simulink model "c00006M_harness"  (R2018a)
settings: Solver=FixedStepAuto  StartTime=0.0  StopTime=300  FixedStep=0.1  RelTol=1e-3
undefined symbols (not defined in the file): A1, hmax, PriorityTank, R1, R2, sigbuilder_block, TempThreshold
(part 5 of 66)

== system c00006M_harness/Eval85 ==
  In2 : Inport
  In3 : Inport  Port=2
  Constant1 : Constant
  Data Type Conversion1 : DataTypeConversion
  Data Type Conversion2 : DataTypeConversion
  Memory2 : Memory  InitialCondition=1
  Memory3 : Memory  InitialCondition=1
  MinMax : MinMax  Inputs=3
  MinMax2 : MinMax  Inputs=2
  MinMax3 : MinMax  Inputs=2
  ROOut2 : RelationalOperator  Operator===  OutDataTypeStr=boolean  RndMeth=Simplest
  ROOut3 : RelationalOperator  Operator===  OutDataTypeStr=boolean  RndMeth=Simplest
  Out1 : Outport
  wires:
  Data Type Conversion2/1 -> MinMax3/1
  Data Type Conversion1/1 -> MinMax2/1
  MinMax2/1 -> MinMax/2, Memory2/1
  Memory2/1 -> MinMax2/2
  Memory3/1 -> MinMax3/2
  ROOut2/1 -> Data Type Conversion1/1
  ROOut3/1 -> Data Type Conversion2/1
  MinMax3/1 -> Memory3/1, MinMax/3
  [out2] -> ROOut2/2
  In2/1 -> ROOut2/1
  In3/1 -> ROOut3/1
  [out3] -> ROOut3/2
  MinMax/1 -> Out1/1
  Constant1/1 -> MinMax/1

== system c00006M_harness/Eval86 ==
  In2 : Inport
  In3 : Inport  Port=2
  Constant1 : Constant
  Data Type Conversion1 : DataTypeConversion
  Data Type Conversion2 : DataTypeConversion
  Memory2 : Memory  InitialCondition=1
  Memory3 : Memory  InitialCondition=1
  MinMax : MinMax  Inputs=3
  MinMax2 : MinMax  Inputs=2
  MinMax3 : MinMax  Inputs=2
  ROOut2 : RelationalOperator  Operator===  OutDataTypeStr=boolean  RndMeth=Simplest
  ROOut3 : RelationalOperator  Operator===  OutDataTypeStr=boolean  RndMeth=Simplest
  Out1 : Outport
  wires:
  Data Type Conversion2/1 -> MinMax3/1
  Data Type Conversion1/1 -> MinMax2/1
  MinMax2/1 -> MinMax/2, Memory2/1
  Memory2/1 -> MinMax2/2
  Memory3/1 -> MinMax3/2
  ROOut2/1 -> Data Type Conversion1/1
  ROOut3/1 -> Data Type Conversion2/1
  MinMax3/1 -> Memory3/1, MinMax/3
  [out2] -> ROOut2/2
  In2/1 -> ROOut2/1
  In3/1 -> ROOut3/1
  [out3] -> ROOut3/2
  MinMax/1 -> Out1/1
  Constant1/1 -> MinMax/1

== system c00006M_harness/Eval87 ==
  In2 : Inport
  In3 : Inport  Port=2
  Constant1 : Constant
  Data Type Conversion1 : DataTypeConversion
  Data Type Conversion2 : DataTypeConversion
  Memory2 : Memory  InitialCondition=1
  Memory3 : Memory  InitialCondition=1
  MinMax : MinMax  Inputs=3
  MinMax2 : MinMax  Inputs=2
  MinMax3 : MinMax  Inputs=2
  ROOut2 : RelationalOperator  Operator===  OutDataTypeStr=boolean  RndMeth=Simplest
  ROOut3 : RelationalOperator  Operator===  OutDataTypeStr=boolean  RndMeth=Simplest
  Out1 : Outport
  wires:
  Data Type Conversion2/1 -> MinMax3/1
  Data Type Conversion1/1 -> MinMax2/1
  MinMax2/1 -> MinMax/2, Memory2/1
  Memory2/1 -> MinMax2/2
  Memory3/1 -> MinMax3/2
  ROOut2/1 -> Data Type Conversion1/1
  ROOut3/1 -> Data Type Conversion2/1
  MinMax3/1 -> Memory3/1, MinMax/3
  [out2] -> ROOut2/2
  In2/1 -> ROOut2/1
  In3/1 -> ROOut3/1
  [out3] -> ROOut3/2
  MinMax/1 -> Out1/1
  Constant1/1 -> MinMax/1

== system c00006M_harness/Eval88 ==
  In2 : Inport
  In3 : Inport  Port=2
  Constant1 : Constant
  Data Type Conversion1 : DataTypeConversion
  Data Type Conversion2 : DataTypeConversion
  Memory2 : Memory  InitialCondition=1
  Memory3 : Memory  InitialCondition=1
  MinMax : MinMax  Inputs=3
  MinMax2 : MinMax  Inputs=2
  MinMax3 : MinMax  Inputs=2
  ROOut2 : RelationalOperator  Operator===  OutDataTypeStr=boolean  RndMeth=Simplest
  ROOut3 : RelationalOperator  Operator===  OutDataTypeStr=boolean  RndMeth=Simplest
  Out1 : Outport
  wires:
  Data Type Conversion2/1 -> MinMax3/1
  Data Type Conversion1/1 -> MinMax2/1
  MinMax2/1 -> MinMax/2, Memory2/1
  Memory2/1 -> MinMax2/2
  Memory3/1 -> MinMax3/2
  ROOut2/1 -> Data Type Conversion1/1
  ROOut3/1 -> Data Type Conversion2/1
  MinMax3/1 -> Memory3/1, MinMax/3
  [out2] -> ROOut2/2
  In2/1 -> ROOut2/1
  In3/1 -> ROOut3/1
  [out3] -> ROOut3/2
  MinMax/1 -> Out1/1
  Constant1/1 -> MinMax/1

== system c00006M_harness/Eval89 ==
  In2 : Inport
  In3 : Inport  Port=2
  Constant1 : Constant
  Data Type Conversion1 : DataTypeConversion
  Data Type Conversion2 : DataTypeConversion
  Memory2 : Memory  InitialCondition=1
  Memory3 : Memory  InitialCondition=1
  MinMax : MinMax  Inputs=3
  MinMax2 : MinMax  Inputs=2
  MinMax3 : MinMax  Inputs=2
  ROOut2 : RelationalOperator  Operator===  OutDataTypeStr=boolean  RndMeth=Simplest
  ROOut3 : RelationalOperator  Operator===  OutDataTypeStr=boolean  RndMeth=Simplest
  Out1 : Outport
  wires:
  Data Type Conversion2/1 -> MinMax3/1
  Data Type Conversion1/1 -> MinMax2/1
  MinMax2/1 -> MinMax/2, Memory2/1
  Memory2/1 -> MinMax2/2
  Memory3/1 -> MinMax3/2
  ROOut2/1 -> Data Type Conversion1/1
  ROOut3/1 -> Data Type Conversion2/1
  MinMax3/1 -> Memory3/1, MinMax/3
  [out2] -> ROOut2/2
  In2/1 -> ROOut2/1
  In3/1 -> ROOut3/1
  [out3] -> ROOut3/2
  MinMax/1 -> Out1/1
  Constant1/1 -> MinMax/1

== system c00006M_harness/Eval90 ==
  In2 : Inport
  In3 : Inport  Port=2
  Constant1 : Constant
  Data Type Conversion1 : DataTypeConversion
  Data Type Conversion2 : DataTypeConversion
  Memory2 : Memory  InitialCondition=1
  Memory3 : Memory  InitialCondition=1
  MinMax : MinMax  Inputs=3
  MinMax2 : MinMax  Inputs=2
  MinMax3 : MinMax  Inputs=2
  ROOut2 : RelationalOperator  Operator===  OutDataTypeStr=boolean  RndMeth=Simplest
  ROOut3 : RelationalOperator  Operator===  OutDataTypeStr=boolean  RndMeth=Simplest
  Out1 : Outport
  wires:
  Data Type Conversion2/1 -> MinMax3/1
  Data Type Conversion1/1 -> MinMax2/1
  MinMax2/1 -> MinMax/2, Memory2/1
  Memory2/1 -> MinMax2/2
  Memory3/1 -> MinMax3/2
  ROOut2/1 -> Data Type Conversion1/1
  ROOut3/1 -> Data Type Conversion2/1
  MinMax3/1 -> Memory3/1, MinMax/3
  [out2] -> ROOut2/2
  In2/1 -> ROOut2/1
  In3/1 -> ROOut3/1
  [out3] -> ROOut3/2
  MinMax/1 -> Out1/1
  Constant1/1 -> MinMax/1

== system c00006M_harness/Eval91 ==
  In2 : Inport
  In3 : Inport  Port=2
  Constant1 : Constant
  Data Type Conversion1 : DataTypeConversion
  Data Type Conversion2 : DataTypeConversion
  Memory2 : Memory  InitialCondition=1
  Memory3 : Memory  InitialCondition=1
  MinMax : MinMax  Inputs=3
  MinMax2 : MinMax  Inputs=2
  MinMax3 : MinMax  Inputs=2
  ROOut2 : RelationalOperator  Operator===  OutDataTypeStr=boolean  RndMeth=Simplest
  ROOut3 : RelationalOperator  Operator===  OutDataTypeStr=boolean  RndMeth=Simplest
  Out1 : Outport
  wires:
  Data Type Conversion2/1 -> MinMax3/1
  Data Type Conversion1/1 -> MinMax2/1
  MinMax2/1 -> MinMax/2, Memory2/1
  Memory2/1 -> MinMax2/2
  Memory3/1 -> MinMax3/2
  ROOut2/1 -> Data Type Conversion1/1
  ROOut3/1 -> Data Type Conversion2/1
  MinMax3/1 -> Memory3/1, MinMax/3
  [out2] -> ROOut2/2
  In2/1 -> ROOut2/1
  In3/1 -> ROOut3/1
  [out3] -> ROOut3/2
  MinMax/1 -> Out1/1
  Constant1/1 -> MinMax/1

== system c00006M_harness/Eval92 ==
  In2 : Inport
  In3 : Inport  Port=2
  Constant1 : Constant
  Data Type Conversion1 : DataTypeConversion
  Data Type Conversion2 : DataTypeConversion
  Memory2 : Memory  InitialCondition=1
  Memory3 : Memory  InitialCondition=1
  MinMax : MinMax  Inputs=3
  MinMax2 : MinMax  Inputs=2
  MinMax3 : MinMax  Inputs=2
  ROOut2 : RelationalOperator  Operator===  OutDataTypeStr=boolean  RndMeth=Simplest
  ROOut3 : RelationalOperator  Operator===  OutDataTypeStr=boolean  RndMeth=Simplest
  Out1 : Outport
  wires:
  Data Type Conversion2/1 -> MinMax3/1
  Data Type Conversion1/1 -> MinMax2/1
  MinMax2/1 -> MinMax/2, Memory2/1
  Memory2/1 -> MinMax2/2
  Memory3/1 -> MinMax3/2
  ROOut2/1 -> Data Type Conversion1/1
  ROOut3/1 -> Data Type Conversion2/1
  MinMax3/1 -> Memory3/1, MinMax/3
  [out2] -> ROOut2/2
  In2/1 -> ROOut2/1
  In3/1 -> ROOut3/1
  [out3] -> ROOut3/2
  MinMax/1 -> Out1/1
  Constant1/1 -> MinMax/1

== system c00006M_harness/Eval93 ==
  In2 : Inport
  In3 : Inport  Port=2
  Constant1 : Constant
  Data Type Conversion1 : DataTypeConversion
  Data Type Conversion2 : DataTypeConversion
  Memory2 : Memory  InitialCondition=1
  Memory3 : Memory  InitialCondition=1
  MinMax : MinMax  Inputs=3
  MinMax2 : MinMax  Inputs=2
  MinMax3 : MinMax  Inputs=2
  ROOut2 : RelationalOperator  Operator===  OutDataTypeStr=boolean  RndMeth=Simplest
  ROOut3 : RelationalOperator  Operator===  OutDataTypeStr=boolean  RndMeth=Simplest
  Out1 : Outport
  wires:
  Data Type Conversion2/1 -> MinMax3/1
  Data Type Conversion1/1 -> MinMax2/1
  MinMax2/1 -> MinMax/2, Memory2/1
  Memory2/1 -> MinMax2/2
  Memory3/1 -> MinMax3/2
  ROOut2/1 -> Data Type Conversion1/1
  ROOut3/1 -> Data Type Conversion2/1
  MinMax3/1 -> Memory3/1, MinMax/3
  [out2] -> ROOut2/2
  In2/1 -> ROOut2/1
  In3/1 -> ROOut3/1
  [out3] -> ROOut3/2
  MinMax/1 -> Out1/1
  Constant1/1 -> MinMax/1

== system c00006M_harness/Eval94 ==
  In2 : Inport
  In3 : Inport  Port=2
  Constant1 : Constant
  Data Type Conversion1 : DataTypeConversion
  Data Type Conversion2 : DataTypeConversion
  Memory2 : Memory  InitialCondition=1
  Memory3 : Memory  InitialCondition=1
  MinMax : MinMax  Inputs=3
  MinMax2 : MinMax  Inputs=2
  MinMax3 : MinMax  Inputs=2
  ROOut2 : RelationalOperator  Operator===  OutDataTypeStr=boolean  RndMeth=Simplest
  ROOut3 : RelationalOperator  Operator===  OutDataTypeStr=boolean  RndMeth=Simplest
  Out1 : Outport
  wires:
  Data Type Conversion2/1 -> MinMax3/1
  Data Type Conversion1/1 -> MinMax2/1
  MinMax2/1 -> MinMax/2, Memory2/1
  Memory2/1 -> MinMax2/2
  Memory3/1 -> MinMax3/2
  ROOut2/1 -> Data Type Conversion1/1
  ROOut3/1 -> Data Type Conversion2/1
  MinMax3/1 -> Memory3/1, MinMax/3
  [out2] -> ROOut2/2
  In2/1 -> ROOut2/1
  In3/1 -> ROOut3/1
  [out3] -> ROOut3/2
  MinMax/1 -> Out1/1
  Constant1/1 -> MinMax/1

== system c00006M_harness/Eval95 ==
  In2 : Inport
  In3 : Inport  Port=2
  Constant1 : Constant
  Data Type Conversion1 : DataTypeConversion
  Data Type Conversion2 : DataTypeConversion
  Memory2 : Memory  InitialCondition=1
  Memory3 : Memory  InitialCondition=1
  MinMax : MinMax  Inputs=3
  MinMax2 : MinMax  Inputs=2
  MinMax3 : MinMax  Inputs=2
  ROOut2 : RelationalOperator  Operator===  OutDataTypeStr=boolean  RndMeth=Simplest
  ROOut3 : RelationalOperator  Operator===  OutDataTypeStr=boolean  RndMeth=Simplest
  Out1 : Outport
  wires:
  Data Type Conversion2/1 -> MinMax3/1
  Data Type Conversion1/1 -> MinMax2/1
  MinMax2/1 -> MinMax/2, Memory2/1
  Memory2/1 -> MinMax2/2
  Memory3/1 -> MinMax3/2
  ROOut2/1 -> Data Type Conversion1/1
  ROOut3/1 -> Data Type Conversion2/1
  MinMax3/1 -> Memory3/1, MinMax/3
  [out2] -> ROOut2/2
  In2/1 -> ROOut2/1
  In3/1 -> ROOut3/1
  [out3] -> ROOut3/2
  MinMax/1 -> Out1/1
  Constant1/1 -> MinMax/1

== system c00006M_harness/Eval96 ==
  In2 : Inport
  In3 : Inport  Port=2
  Constant1 : Constant
  Data Type Conversion1 : DataTypeConversion
  Data Type Conversion2 : DataTypeConversion
  Memory2 : Memory  InitialCondition=1
  Memory3 : Memory  InitialCondition=1
  MinMax : MinMax  Inputs=3
  MinMax2 : MinMax  Inputs=2
  MinMax3 : MinMax  Inputs=2
  ROOut2 : RelationalOperator  Operator===  OutDataTypeStr=boolean  RndMeth=Simplest
  ROOut3 : RelationalOperator  Operator===  OutDataTypeStr=boolean  RndMeth=Simplest
  Out1 : Outport
  wires:
  Data Type Conversion2/1 -> MinMax3/1
  Data Type Conversion1/1 -> MinMax2/1
  MinMax2/1 -> MinMax/2, Memory2/1
  Memory2/1 -> MinMax2/2
  Memory3/1 -> MinMax3/2
  ROOut2/1 -> Data Type Conversion1/1
  ROOut3/1 -> Data Type Conversion2/1
  MinMax3/1 -> Memory3/1, MinMax/3
  [out2] -> ROOut2/2
  In2/1 -> ROOut2/1
  In3/1 -> ROOut3/1
  [out3] -> ROOut3/2
  MinMax/1 -> Out1/1
  Constant1/1 -> MinMax/1

== system c00006M_harness/Eval97 ==
  In2 : Inport
  In3 : Inport  Port=2
  Constant1 : Constant
  Data Type Conversion1 : DataTypeConversion
  Data Type Conversion2 : DataTypeConversion
  Memory2 : Memory  InitialCondition=1
  Memory3 : Memory  InitialCondition=1
  MinMax : MinMax  Inputs=3
  MinMax2 : MinMax  Inputs=2
  MinMax3 : MinMax  Inputs=2
  ROOut2 : RelationalOperator  Operator===  OutDataTypeStr=boolean  RndMeth=Simplest
  ROOut3 : RelationalOperator  Operator===  OutDataTypeStr=boolean  RndMeth=Simplest
  Out1 : Outport
  wires:
  Data Type Conversion2/1 -> MinMax3/1
  Data Type Conversion1/1 -> MinMax2/1
  MinMax2/1 -> MinMax/2, Memory2/1
  Memory2/1 -> MinMax2/2
  Memory3/1 -> MinMax3/2
  ROOut2/1 -> Data Type Conversion1/1
  ROOut3/1 -> Data Type Conversion2/1
  MinMax3/1 -> Memory3/1, MinMax/3
  [out2] -> ROOut2/2
  In2/1 -> ROOut2/1
  In3/1 -> ROOut3/1
  [out3] -> ROOut3/2
  MinMax/1 -> Out1/1
  Constant1/1 -> MinMax/1

== system c00006M_harness/Eval98 ==
  In2 : Inport
  In3 : Inport  Port=2
  Constant1 : Constant
  Data Type Conversion1 : DataTypeConversion
  Data Type Conversion2 : DataTypeConversion
  Memory2 : Memory  InitialCondition=1
  Memory3 : Memory  InitialCondition=1
  MinMax : MinMax  Inputs=3
  MinMax2 : MinMax  Inputs=2
  MinMax3 : MinMax  Inputs=2
  ROOut2 : RelationalOperator  Operator===  OutDataTypeStr=boolean  RndMeth=Simplest
  ROOut3 : RelationalOperator  Operator===  OutDataTypeStr=boolean  RndMeth=Simplest
  Out1 : Outport
  wires:
  Data Type Conversion2/1 -> MinMax3/1
  Data Type Conversion1/1 -> MinMax2/1
  MinMax2/1 -> MinMax/2, Memory2/1
  Memory2/1 -> MinMax2/2
  Memory3/1 -> MinMax3/2
  ROOut2/1 -> Data Type Conversion1/1
  ROOut3/1 -> Data Type Conversion2/1
  MinMax3/1 -> Memory3/1, MinMax/3
  [out2] -> ROOut2/2
  In2/1 -> ROOut2/1
  In3/1 -> ROOut3/1
  [out3] -> ROOut3/2
  MinMax/1 -> Out1/1
  Constant1/1 -> MinMax/1

== system c00006M_harness/Eval99 ==
  In2 : Inport
  In3 : Inport  Port=2
  Constant1 : Constant
  Data Type Conversion1 : DataTypeConversion
  Data Type Conversion2 : DataTypeConversion
  Memory2 : Memory  InitialCondition=1
  Memory3 : Memory  InitialCondition=1
  MinMax : MinMax  Inputs=3
  MinMax2 : MinMax  Inputs=2
  MinMax3 : MinMax  Inputs=2
  ROOut2 : RelationalOperator  Operator===  OutDataTypeStr=boolean  RndMeth=Simplest
  ROOut3 : RelationalOperator  Operator===  OutDataTypeStr=boolean  RndMeth=Simplest
  Out1 : Outport
  wires:
  Data Type Conversion2/1 -> MinMax3/1
  Data Type Conversion1/1 -> MinMax2/1
  MinMax2/1 -> MinMax/2, Memory2/1
  Memory2/1 -> MinMax2/2
  Memory3/1 -> MinMax3/2
  ROOut2/1 -> Data Type Conversion1/1
  ROOut3/1 -> Data Type Conversion2/1
  MinMax3/1 -> Memory3/1, MinMax/3
  [out2] -> ROOut2/2
  In2/1 -> ROOut2/1
  In3/1 -> ROOut3/1
  [out3] -> ROOut3/2
  MinMax/1 -> Out1/1
  Constant1/1 -> MinMax/1

== system c00006M_harness/Inputs ==
  Demux : Demux  Tag=STV Demux  Outputs=12
  FromWs : FromWorkspace  Tag=STV FromWs  VariableName=tuvar  SampleTime=0
  CT2 : Outport  Tag=STV Outport
  F2 : Outport  Tag=STV Outport  Port=2
  E2 : Outport  Tag=STV Outport  Port=3
  MR2 : Outport  Tag=STV Outport  Port=4
  T2 : Outport  Tag=STV Outport  Port=5
  EB2 : Outport  Tag=STV Outport  Port=6
  CT3 : Outport  Tag=STV Outport  Port=7
  F3 : Outport  Tag=STV Outport  Port=8
  E3 : Outport  Tag=STV Outport  Port=9
  MR3 : Outport  Tag=STV Outport  Port=10
  T3 : Outport  Tag=STV Outport  Port=11
  EB3 : Outport  Tag=STV Outport  Port=12
  wires:
  Demux/12 -> EB3/1
  Demux/11 -> T3/1
  Demux/10 -> MR3/1
  Demux/9 -> E3/1
  Demux/8 -> F3/1
  Demux/7 -> CT3/1
  Demux/6 -> EB2/1
  Demux/5 -> T2/1
  Demux/4 -> MR2/1
  Demux/3 -> E2/1
  Demux/2 -> F2/1
  Demux/1 -> CT2/1
  FromWs/1 -> Demux/1

== system c00006M_harness/M062 ==
  note: VALUES
      | ---------------------------------
      | ControlType = 1 | 2 | 3
      | FillTank = 0 | 1
      | EmptyTank = 0 | 1
      | ManualReference between 0 and 1
      | Tempreature between 0 and 100
      | EmergencyButton = 0 | 1
      | LiquidLevel between 0 and 1 (hmax)
  note: Inputs For Tank2
  note: NAMES
      | --------------------------------------------
      | CT1 = ControlType Tank 1
      | F1 = Fill Tank 1
      | E1 = Empty Tank 1
      | MR1 = Manual Reference Tank1
      | T1 = Temperature Tank 1
      | EB1 = Emergency Button Tank 1
      | LL1 = Liquid Level 1
  note: Inputs For Tank3
  note: Inputs For Tank1
  CT2 : Inport
  F2 : Inport  Port=2
  E2 : Inport  Port=3
  MR2 : Inport  Port=4
  T2 : Inport  Port=5
  EB2 : Inport  Port=6
  CT3 : Inport  Port=7
  F3 : Inport  Port=8
  E3 : Inport  Port=9
  MR3 : Inport  Port=10
  T3 : Inport  Port=11
  EB3 : Inport  Port=12
  Tank2 : Subsystem
  Tank3 : Subsystem
  LL2 : Outport
  LL3 : Outport  Port=2
  wires:
  Tank2/1(LL2) -> LL2/1, Tank3/7(LL2)
  Tank3/1(LL3) -> LL3/1, Tank2/7(LL3)
  EB2/1 -> Tank2/6(EB2)
  MR3/1 -> Tank3/4(MR3)
  CT2/1 -> Tank2/1(CT2)
  F2/1 -> Tank2/2(F2)
  E3/1 -> Tank3/3(E3)
  E2/1 -> Tank2/3(E2)
  T2/1 -> Tank2/5(T2)
  CT3/1 -> Tank3/1(CT3)
  F3/1 -> Tank3/2(F3)
  EB3/1 -> Tank3/6(EB3)
  T3/1 -> Tank3/5(T3)
  MR2/1 -> Tank2/4(MR2)

== system c00006M_harness/M063 ==
  note: VALUES
      | ---------------------------------
      | ControlType = 1 | 2 | 3
      | FillTank = 0 | 1
      | EmptyTank = 0 | 1
      | ManualReference between 0 and 1
      | Tempreature between 0 and 100
      | EmergencyButton = 0 | 1
      | LiquidLevel between 0 and 1 (hmax)
  note: Inputs For Tank2
  note: NAMES
      | --------------------------------------------
      | CT1 = ControlType Tank 1
      | F1 = Fill Tank 1
      | E1 = Empty Tank 1
      | MR1 = Manual Reference Tank1
      | T1 = Temperature Tank 1
      | EB1 = Emergency Button Tank 1
      | LL1 = Liquid Level 1
  note: Inputs For Tank3
  note: Inputs For Tank1
  CT2 : Inport
  F2 : Inport  Port=2
  E2 : Inport  Port=3
  MR2 : Inport  Port=4
  T2 : Inport  Port=5
  EB2 : Inport  Port=6
  CT3 : Inport  Port=7
  F3 : Inport  Port=8
  E3 : Inport  Port=9
  MR3 : Inport  Port=10
  T3 : Inport  Port=11
  EB3 : Inport  Port=12
  Tank2 : Subsystem
  Tank3 : Subsystem
  LL2 : Outport
  LL3 : Outport  Port=2
  wires:
  Tank2/1(LL2) -> LL2/1, Tank3/7(LL2)
  Tank3/1(LL3) -> LL3/1, Tank2/7(LL3)
  EB2/1 -> Tank2/6(EB2)
  MR3/1 -> Tank3/4(MR3)
  CT2/1 -> Tank2/1(CT2)
  F2/1 -> Tank2/2(F2)
  E3/1 -> Tank3/3(E3)
  E2/1 -> Tank2/3(E2)
  T2/1 -> Tank2/5(T2)
  CT3/1 -> Tank3/1(CT3)
  F3/1 -> Tank3/2(F3)
  EB3/1 -> Tank3/6(EB3)
  T3/1 -> Tank3/5(T3)
  MR2/1 -> Tank2/4(MR2)

== system c00006M_harness/M064 ==
  note: VALUES
      | ---------------------------------
      | ControlType = 1 | 2 | 3
      | FillTank = 0 | 1
      | EmptyTank = 0 | 1
      | ManualReference between 0 and 1
      | Tempreature between 0 and 100
      | EmergencyButton = 0 | 1
      | LiquidLevel between 0 and 1 (hmax)
  note: Inputs For Tank2
  note: NAMES
      | --------------------------------------------
      | CT1 = ControlType Tank 1
      | F1 = Fill Tank 1
      | E1 = Empty Tank 1
      | MR1 = Manual Reference Tank1
      | T1 = Temperature Tank 1
      | EB1 = Emergency Button Tank 1
      | LL1 = Liquid Level 1
  note: Inputs For Tank3
  note: Inputs For Tank1
  CT2 : Inport
  F2 : Inport  Port=2
  E2 : Inport  Port=3
  MR2 : Inport  Port=4
  T2 : Inport  Port=5
  EB2 : Inport  Port=6
  CT3 : Inport  Port=7
  F3 : Inport  Port=8
  E3 : Inport  Port=9
  MR3 : Inport  Port=10
  T3 : Inport  Port=11
  EB3 : Inport  Port=12
  Tank2 : Subsystem
  Tank3 : Subsystem
  LL2 : Outport
  LL3 : Outport  Port=2
  wires:
  Tank2/1(LL2) -> LL2/1, Tank3/7(LL2)
  Tank3/1(LL3) -> LL3/1, Tank2/7(LL3)
  EB2/1 -> Tank2/6(EB2)
  MR3/1 -> Tank3/4(MR3)
  CT2/1 -> Tank2/1(CT2)
  F2/1 -> Tank2/2(F2)
  E3/1 -> Tank3/3(E3)
  E2/1 -> Tank2/3(E2)
  T2/1 -> Tank2/5(T2)
  CT3/1 -> Tank3/1(CT3)
  F3/1 -> Tank3/2(F3)
  EB3/1 -> Tank3/6(EB3)
  T3/1 -> Tank3/5(T3)
  MR2/1 -> Tank2/4(MR2)

== system c00006M_harness/M065 ==
  note: VALUES
      | ---------------------------------
      | ControlType = 1 | 2 | 3
      | FillTank = 0 | 1
      | EmptyTank = 0 | 1
      | ManualReference between 0 and 1
      | Tempreature between 0 and 100
      | EmergencyButton = 0 | 1
      | LiquidLevel between 0 and 1 (hmax)
  note: Inputs For Tank2
  note: NAMES
      | --------------------------------------------
      | CT1 = ControlType Tank 1
      | F1 = Fill Tank 1
      | E1 = Empty Tank 1
      | MR1 = Manual Reference Tank1
      | T1 = Temperature Tank 1
      | EB1 = Emergency Button Tank 1
      | LL1 = Liquid Level 1
  note: Inputs For Tank3
  note: Inputs For Tank1
  CT2 : Inport
  F2 : Inport  Port=2
  E2 : Inport  Port=3
  MR2 : Inport  Port=4
  T2 : Inport  Port=5
  EB2 : Inport  Port=6
  CT3 : Inport  Port=7
  F3 : Inport  Port=8
  E3 : Inport  Port=9
  MR3 : Inport  Port=10
  T3 : Inport  Port=11
  EB3 : Inport  Port=12
  Tank2 : Subsystem
  Tank3 : Subsystem
  LL2 : Outport
  LL3 : Outport  Port=2
  wires:
  Tank2/1(LL2) -> LL2/1, Tank3/7(LL2)
  Tank3/1(LL3) -> LL3/1, Tank2/7(LL3)
  EB2/1 -> Tank2/6(EB2)
  MR3/1 -> Tank3/4(MR3)
  CT2/1 -> Tank2/1(CT2)
  F2/1 -> Tank2/2(F2)
  E3/1 -> Tank3/3(E3)
  E2/1 -> Tank2/3(E2)
  T2/1 -> Tank2/5(T2)
  CT3/1 -> Tank3/1(CT3)
  F3/1 -> Tank3/2(F3)
  EB3/1 -> Tank3/6(EB3)
  T3/1 -> Tank3/5(T3)
  MR2/1 -> Tank2/4(MR2)

== system c00006M_harness/M066 ==
  note: VALUES
      | ---------------------------------
      | ControlType = 1 | 2 | 3
      | FillTank = 0 | 1
      | EmptyTank = 0 | 1
      | ManualReference between 0 and 1
      | Tempreature between 0 and 100
      | EmergencyButton = 0 | 1
      | LiquidLevel between 0 and 1 (hmax)
  note: Inputs For Tank2
  note: NAMES
      | --------------------------------------------
      | CT1 = ControlType Tank 1
      | F1 = Fill Tank 1
      | E1 = Empty Tank 1
      | MR1 = Manual Reference Tank1
      | T1 = Temperature Tank 1
      | EB1 = Emergency Button Tank 1
      | LL1 = Liquid Level 1
  note: Inputs For Tank3
  note: Inputs For Tank1
  CT2 : Inport
  F2 : Inport  Port=2
  E2 : Inport  Port=3
  MR2 : Inport  Port=4
  T2 : Inport  Port=5
  EB2 : Inport  Port=6
  CT3 : Inport  Port=7
  F3 : Inport  Port=8
  E3 : Inport  Port=9
  MR3 : Inport  Port=10
  T3 : Inport  Port=11
  EB3 : Inport  Port=12
  Tank2 : Subsystem
  Tank3 : Subsystem
  LL2 : Outport
  LL3 : Outport  Port=2
  wires:
  Tank2/1(LL2) -> LL2/1, Tank3/7(LL2)
  Tank3/1(LL3) -> LL3/1, Tank2/7(LL3)
  EB2/1 -> Tank2/6(EB2)
  MR3/1 -> Tank3/4(MR3)
  CT2/1 -> Tank2/1(CT2)
  F2/1 -> Tank2/2(F2)
  E3/1 -> Tank3/3(E3)
  E2/1 -> Tank2/3(E2)
  T2/1 -> Tank2/5(T2)
  CT3/1 -> Tank3/1(CT3)
  F3/1 -> Tank3/2(F3)
  EB3/1 -> Tank3/6(EB3)
  T3/1 -> Tank3/5(T3)
  MR2/1 -> Tank2/4(MR2)

== system c00006M_harness/M083 ==
  note: VALUES
      | ---------------------------------
      | ControlType = 1 | 2 | 3
      | FillTank = 0 | 1
      | EmptyTank = 0 | 1
      | ManualReference between 0 and 1
      | Tempreature between 0 and 100
      | EmergencyButton = 0 | 1
      | LiquidLevel between 0 and 1 (hmax)
  note: Inputs For Tank2
  note: NAMES
      | --------------------------------------------
      | CT1 = ControlType Tank 1
      | F1 = Fill Tank 1
      | E1 = Empty Tank 1
      | MR1 = Manual Reference Tank1
      | T1 = Temperature Tank 1
      | EB1 = Emergency Button Tank 1
      | LL1 = Liquid Level 1
  note: Inputs For Tank3
  note: Inputs For Tank1
  CT2 : Inport
  F2 : Inport  Port=2
  E2 : Inport  Port=3
  MR2 : Inport  Port=4
  T2 : Inport  Port=5
  EB2 : Inport  Port=6
  CT3 : Inport  Port=7
  F3 : Inport  Port=8
  E3 : Inport  Port=9
  MR3 : Inport  Port=10
  T3 : Inport  Port=11
  EB3 : Inport  Port=12
  Tank2 : Subsystem
  Tank3 : Subsystem
  LL2 : Outport
  LL3 : Outport  Port=2
  wires:
  Tank2/1(LL2) -> LL2/1, Tank3/7(LL2)
  Tank3/1(LL3) -> LL3/1, Tank2/7(LL3)
  EB2/1 -> Tank2/6(EB2)
  MR3/1 -> Tank3/4(MR3)
  CT2/1 -> Tank2/1(CT2)
  F2/1 -> Tank2/2(F2)
  E3/1 -> Tank3/3(E3)
  E2/1 -> Tank2/3(E2)
  T2/1 -> Tank2/5(T2)
  CT3/1 -> Tank3/1(CT3)
  F3/1 -> Tank3/2(F3)
  EB3/1 -> Tank3/6(EB3)
  T3/1 -> Tank3/5(T3)
  MR2/1 -> Tank2/4(MR2)

== system c00006M_harness/M084 ==
  note: VALUES
      | ---------------------------------
      | ControlType = 1 | 2 | 3
      | FillTank = 0 | 1
      | EmptyTank = 0 | 1
      | ManualReference between 0 and 1
      | Tempreature between 0 and 100
      | EmergencyButton = 0 | 1
      | LiquidLevel between 0 and 1 (hmax)
  note: Inputs For Tank2
  note: NAMES
      | --------------------------------------------
      | CT1 = ControlType Tank 1
      | F1 = Fill Tank 1
      | E1 = Empty Tank 1
      | MR1 = Manual Reference Tank1
      | T1 = Temperature Tank 1
      | EB1 = Emergency Button Tank 1
      | LL1 = Liquid Level 1
  note: Inputs For Tank3
  note: Inputs For Tank1
  CT2 : Inport
  F2 : Inport  Port=2
  E2 : Inport  Port=3
  MR2 : Inport  Port=4
  T2 : Inport  Port=5
  EB2 : Inport  Port=6
  CT3 : Inport  Port=7
  F3 : Inport  Port=8
  E3 : Inport  Port=9
  MR3 : Inport  Port=10
  T3 : Inport  Port=11
  EB3 : Inport  Port=12
  Tank2 : Subsystem
  Tank3 : Subsystem
  LL2 : Outport
  LL3 : Outport  Port=2
  wires:
  Tank2/1(LL2) -> LL2/1, Tank3/7(LL2)
  Tank3/1(LL3) -> LL3/1, Tank2/7(LL3)
  EB2/1 -> Tank2/6(EB2)
  MR3/1 -> Tank3/4(MR3)
  CT2/1 -> Tank2/1(CT2)
  F2/1 -> Tank2/2(F2)
  E3/1 -> Tank3/3(E3)
  E2/1 -> Tank2/3(E2)
  T2/1 -> Tank2/5(T2)
  CT3/1 -> Tank3/1(CT3)
  F3/1 -> Tank3/2(F3)
  EB3/1 -> Tank3/6(EB3)
  T3/1 -> Tank3/5(T3)
  MR2/1 -> Tank2/4(MR2)

== system c00006M_harness/M085 ==
  note: VALUES
      | ---------------------------------
      | ControlType = 1 | 2 | 3
      | FillTank = 0 | 1
      | EmptyTank = 0 | 1
      | ManualReference between 0 and 1
      | Tempreature between 0 and 100
      | EmergencyButton = 0 | 1
      | LiquidLevel between 0 and 1 (hmax)
  note: Inputs For Tank2
  note: NAMES
      | --------------------------------------------
      | CT1 = ControlType Tank 1
      | F1 = Fill Tank 1
      | E1 = Empty Tank 1
      | MR1 = Manual Reference Tank1
      | T1 = Temperature Tank 1
      | EB1 = Emergency Button Tank 1
      | LL1 = Liquid Level 1
  note: Inputs For Tank3
  note: Inputs For Tank1
  CT2 : Inport
  F2 : Inport  Port=2
  E2 : Inport  Port=3
  MR2 : Inport  Port=4
  T2 : Inport  Port=5
  EB2 : Inport  Port=6
  CT3 : Inport  Port=7
  F3 : Inport  Port=8
  E3 : Inport  Port=9
  MR3 : Inport  Port=10
  T3 : Inport  Port=11
  EB3 : Inport  Port=12
  Tank2 : Subsystem
  Tank3 : Subsystem
  LL2 : Outport
  LL3 : Outport  Port=2
  wires:
  Tank2/1(LL2) -> LL2/1, Tank3/7(LL2)
  Tank3/1(LL3) -> LL3/1, Tank2/7(LL3)
  EB2/1 -> Tank2/6(EB2)
  MR3/1 -> Tank3/4(MR3)
  CT2/1 -> Tank2/1(CT2)
  F2/1 -> Tank2/2(F2)
  E3/1 -> Tank3/3(E3)
  E2/1 -> Tank2/3(E2)
  T2/1 -> Tank2/5(T2)
  CT3/1 -> Tank3/1(CT3)
  F3/1 -> Tank3/2(F3)
  EB3/1 -> Tank3/6(EB3)
  T3/1 -> Tank3/5(T3)
  MR2/1 -> Tank2/4(MR2)

== system c00006M_harness/M086 ==
  note: VALUES
      | ---------------------------------
      | ControlType = 1 | 2 | 3
      | FillTank = 0 | 1
      | EmptyTank = 0 | 1
      | ManualReference between 0 and 1
      | Tempreature between 0 and 100
      | EmergencyButton = 0 | 1
      | LiquidLevel between 0 and 1 (hmax)
  note: Inputs For Tank2
  note: NAMES
      | --------------------------------------------
      | CT1 = ControlType Tank 1
      | F1 = Fill Tank 1
      | E1 = Empty Tank 1
      | MR1 = Manual Reference Tank1
      | T1 = Temperature Tank 1
      | EB1 = Emergency Button Tank 1
      | LL1 = Liquid Level 1
  note: Inputs For Tank3
  note: Inputs For Tank1
  CT2 : Inport
  F2 : Inport  Port=2
  E2 : Inport  Port=3
  MR2 : Inport  Port=4
  T2 : Inport  Port=5
  EB2 : Inport  Port=6
  CT3 : Inport  Port=7
  F3 : Inport  Port=8
  E3 : Inport  Port=9
  MR3 : Inport  Port=10
  T3 : Inport  Port=11
  EB3 : Inport  Port=12
  Tank2 : Subsystem
  Tank3 : Subsystem
  LL2 : Outport
  LL3 : Outport  Port=2
  wires:
  Tank2/1(LL2) -> LL2/1, Tank3/7(LL2)
  Tank3/1(LL3) -> LL3/1, Tank2/7(LL3)
  EB2/1 -> Tank2/6(EB2)
  MR3/1 -> Tank3/4(MR3)
  CT2/1 -> Tank2/1(CT2)
  F2/1 -> Tank2/2(F2)
  E3/1 -> Tank3/3(E3)
  E2/1 -> Tank2/3(E2)
  T2/1 -> Tank2/5(T2)
  CT3/1 -> Tank3/1(CT3)
  F3/1 -> Tank3/2(F3)
  EB3/1 -> Tank3/6(EB3)
  T3/1 -> Tank3/5(T3)
  MR2/1 -> Tank2/4(MR2)

== system c00006M_harness/M087 ==
  note: VALUES
      | ---------------------------------
      | ControlType = 1 | 2 | 3
      | FillTank = 0 | 1
      | EmptyTank = 0 | 1
      | ManualReference between 0 and 1
      | Tempreature between 0 and 100
      | EmergencyButton = 0 | 1
      | LiquidLevel between 0 and 1 (hmax)
  note: Inputs For Tank2
  note: NAMES
      | --------------------------------------------
      | CT1 = ControlType Tank 1
      | F1 = Fill Tank 1
      | E1 = Empty Tank 1
      | MR1 = Manual Reference Tank1
      | T1 = Temperature Tank 1
      | EB1 = Emergency Button Tank 1
      | LL1 = Liquid Level 1
  note: Inputs For Tank3
  note: Inputs For Tank1
  CT2 : Inport
  F2 : Inport  Port=2
  E2 : Inport  Port=3
  MR2 : Inport  Port=4
  T2 : Inport  Port=5
  EB2 : Inport  Port=6
  CT3 : Inport  Port=7
  F3 : Inport  Port=8
  E3 : Inport  Port=9
  MR3 : Inport  Port=10
  T3 : Inport  Port=11
  EB3 : Inport  Port=12
  Tank2 : Subsystem
  Tank3 : Subsystem
  LL2 : Outport
  LL3 : Outport  Port=2
  wires:
  Tank2/1(LL2) -> LL2/1, Tank3/7(LL2)
  Tank3/1(LL3) -> LL3/1, Tank2/7(LL3)
  EB2/1 -> Tank2/6(EB2)
  MR3/1 -> Tank3/4(MR3)
  CT2/1 -> Tank2/1(CT2)
  F2/1 -> Tank2/2(F2)
  E3/1 -> Tank3/3(E3)
  E2/1 -> Tank2/3(E2)
  T2/1 -> Tank2/5(T2)
  CT3/1 -> Tank3/1(CT3)
  F3/1 -> Tank3/2(F3)
  EB3/1 -> Tank3/6(EB3)
  T3/1 -> Tank3/5(T3)
  MR2/1 -> Tank2/4(MR2)

== system c00006M_harness/M088 ==
  note: VALUES
      | ---------------------------------
      | ControlType = 1 | 2 | 3
      | FillTank = 0 | 1
      | EmptyTank = 0 | 1
      | ManualReference between 0 and 1
      | Tempreature between 0 and 100
      | EmergencyButton = 0 | 1
      | LiquidLevel between 0 and 1 (hmax)
  note: Inputs For Tank2
  note: NAMES
      | --------------------------------------------
      | CT1 = ControlType Tank 1
      | F1 = Fill Tank 1
      | E1 = Empty Tank 1
      | MR1 = Manual Reference Tank1
      | T1 = Temperature Tank 1
      | EB1 = Emergency Button Tank 1
      | LL1 = Liquid Level 1
  note: Inputs For Tank3
  note: Inputs For Tank1
  CT2 : Inport
  F2 : Inport  Port=2
  E2 : Inport  Port=3
  MR2 : Inport  Port=4
  T2 : Inport  Port=5
  EB2 : Inport  Port=6
  CT3 : Inport  Port=7
  F3 : Inport  Port=8
  E3 : Inport  Port=9
  MR3 : Inport  Port=10
  T3 : Inport  Port=11
  EB3 : Inport  Port=12
  Tank2 : Subsystem
  Tank3 : Subsystem
  LL2 : Outport
  LL3 : Outport  Port=2
  wires:
  Tank2/1(LL2) -> LL2/1, Tank3/7(LL2)
  Tank3/1(LL3) -> LL3/1, Tank2/7(LL3)
  EB2/1 -> Tank2/6(EB2)
  MR3/1 -> Tank3/4(MR3)
  CT2/1 -> Tank2/1(CT2)
  F2/1 -> Tank2/2(F2)
  E3/1 -> Tank3/3(E3)
  E2/1 -> Tank2/3(E2)
  T2/1 -> Tank2/5(T2)
  CT3/1 -> Tank3/1(CT3)
  F3/1 -> Tank3/2(F3)
  EB3/1 -> Tank3/6(EB3)
  T3/1 -> Tank3/5(T3)
  MR2/1 -> Tank2/4(MR2)

== system c00006M_harness/M089 ==
  note: VALUES
      | ---------------------------------
      | ControlType = 1 | 2 | 3
      | FillTank = 0 | 1
      | EmptyTank = 0 | 1
      | ManualReference between 0 and 1
      | Tempreature between 0 and 100
      | EmergencyButton = 0 | 1
      | LiquidLevel between 0 and 1 (hmax)
  note: Inputs For Tank2
  note: NAMES
      | --------------------------------------------
      | CT1 = ControlType Tank 1
      | F1 = Fill Tank 1
      | E1 = Empty Tank 1
      | MR1 = Manual Reference Tank1
      | T1 = Temperature Tank 1
      | EB1 = Emergency Button Tank 1
      | LL1 = Liquid Level 1
  note: Inputs For Tank3
  note: Inputs For Tank1
  CT2 : Inport
  F2 : Inport  Port=2
  E2 : Inport  Port=3
  MR2 : Inport  Port=4
  T2 : Inport  Port=5
  EB2 : Inport  Port=6
  CT3 : Inport  Port=7
  F3 : Inport  Port=8
  E3 : Inport  Port=9
  MR3 : Inport  Port=10
  T3 : Inport  Port=11
  EB3 : Inport  Port=12
  Tank2 : Subsystem
  Tank3 : Subsystem
  LL2 : Outport
  LL3 : Outport  Port=2
  wires:
  Tank2/1(LL2) -> LL2/1, Tank3/7(LL2)
  Tank3/1(LL3) -> LL3/1, Tank2/7(LL3)
  EB2/1 -> Tank2/6(EB2)
  MR3/1 -> Tank3/4(MR3)
  CT2/1 -> Tank2/1(CT2)
  F2/1 -> Tank2/2(F2)
  E3/1 -> Tank3/3(E3)
  E2/1 -> Tank2/3(E2)
  T2/1 -> Tank2/5(T2)
  CT3/1 -> Tank3/1(CT3)
  F3/1 -> Tank3/2(F3)
  EB3/1 -> Tank3/6(EB3)
  T3/1 -> Tank3/5(T3)
  MR2/1 -> Tank2/4(MR2)

== system c00006M_harness/M090 ==
  note: VALUES
      | ---------------------------------
      | ControlType = 1 | 2 | 3
      | FillTank = 0 | 1
      | EmptyTank = 0 | 1
      | ManualReference between 0 and 1
      | Tempreature between 0 and 100
      | EmergencyButton = 0 | 1
      | LiquidLevel between 0 and 1 (hmax)
  note: Inputs For Tank2
  note: NAMES
      | --------------------------------------------
      | CT1 = ControlType Tank 1
      | F1 = Fill Tank 1
      | E1 = Empty Tank 1
      | MR1 = Manual Reference Tank1
      | T1 = Temperature Tank 1
      | EB1 = Emergency Button Tank 1
      | LL1 = Liquid Level 1
  note: Inputs For Tank3
  note: Inputs For Tank1
  CT2 : Inport
  F2 : Inport  Port=2
  E2 : Inport  Port=3
  MR2 : Inport  Port=4
  T2 : Inport  Port=5
  EB2 : Inport  Port=6
  CT3 : Inport  Port=7
  F3 : Inport  Port=8
  E3 : Inport  Port=9
  MR3 : Inport  Port=10
  T3 : Inport  Port=11
  EB3 : Inport  Port=12
  Tank2 : Subsystem
  Tank3 : Subsystem
  LL2 : Outport
  LL3 : Outport  Port=2
  wires:
  Tank2/1(LL2) -> LL2/1, Tank3/7(LL2)
  Tank3/1(LL3) -> LL3/1, Tank2/7(LL3)
  EB2/1 -> Tank2/6(EB2)
  MR3/1 -> Tank3/4(MR3)
  CT2/1 -> Tank2/1(CT2)
  F2/1 -> Tank2/2(F2)
  E3/1 -> Tank3/3(E3)
  E2/1 -> Tank2/3(E2)
  T2/1 -> Tank2/5(T2)
  CT3/1 -> Tank3/1(CT3)
  F3/1 -> Tank3/2(F3)
  EB3/1 -> Tank3/6(EB3)
  T3/1 -> Tank3/5(T3)
  MR2/1 -> Tank2/4(MR2)

== system c00006M_harness/M091 ==
  note: VALUES
      | ---------------------------------
      | ControlType = 1 | 2 | 3
      | FillTank = 0 | 1
      | EmptyTank = 0 | 1
      | ManualReference between 0 and 1
      | Tempreature between 0 and 100
      | EmergencyButton = 0 | 1
      | LiquidLevel between 0 and 1 (hmax)
  note: Inputs For Tank2
  note: NAMES
      | --------------------------------------------
      | CT1 = ControlType Tank 1
      | F1 = Fill Tank 1
      | E1 = Empty Tank 1
      | MR1 = Manual Reference Tank1
      | T1 = Temperature Tank 1
      | EB1 = Emergency Button Tank 1
      | LL1 = Liquid Level 1
  note: Inputs For Tank3
  note: Inputs For Tank1
  CT2 : Inport
  F2 : Inport  Port=2
  E2 : Inport  Port=3
  MR2 : Inport  Port=4
  T2 : Inport  Port=5
  EB2 : Inport  Port=6
  CT3 : Inport  Port=7
  F3 : Inport  Port=8
  E3 : Inport  Port=9
  MR3 : Inport  Port=10
  T3 : Inport  Port=11
  EB3 : Inport  Port=12
  Tank2 : Subsystem
  Tank3 : Subsystem
  LL2 : Outport
  LL3 : Outport  Port=2
  wires:
  Tank2/1(LL2) -> LL2/1, Tank3/7(LL2)
  Tank3/1(LL3) -> LL3/1, Tank2/7(LL3)
  EB2/1 -> Tank2/6(EB2)
  MR3/1 -> Tank3/4(MR3)
  CT2/1 -> Tank2/1(CT2)
  F2/1 -> Tank2/2(F2)
  E3/1 -> Tank3/3(E3)
  E2/1 -> Tank2/3(E2)
  T2/1 -> Tank2/5(T2)
  CT3/1 -> Tank3/1(CT3)
  F3/1 -> Tank3/2(F3)
  EB3/1 -> Tank3/6(EB3)
  T3/1 -> Tank3/5(T3)
  MR2/1 -> Tank2/4(MR2)

== system c00006M_harness/M092 ==
  note: VALUES
      | ---------------------------------
      | ControlType = 1 | 2 | 3
      | FillTank = 0 | 1
      | EmptyTank = 0 | 1
      | ManualReference between 0 and 1
      | Tempreature between 0 and 100
      | EmergencyButton = 0 | 1
      | LiquidLevel between 0 and 1 (hmax)
  note: Inputs For Tank2
  note: NAMES
      | --------------------------------------------
      | CT1 = ControlType Tank 1
      | F1 = Fill Tank 1
      | E1 = Empty Tank 1
      | MR1 = Manual Reference Tank1
      | T1 = Temperature Tank 1
      | EB1 = Emergency Button Tank 1
      | LL1 = Liquid Level 1
  note: Inputs For Tank3
  note: Inputs For Tank1
  CT2 : Inport
  F2 : Inport  Port=2
  E2 : Inport  Port=3
  MR2 : Inport  Port=4
  T2 : Inport  Port=5
  EB2 : Inport  Port=6
  CT3 : Inport  Port=7
  F3 : Inport  Port=8
  E3 : Inport  Port=9
  MR3 : Inport  Port=10
  T3 : Inport  Port=11
  EB3 : Inport  Port=12
  Tank2 : Subsystem
  Tank3 : Subsystem
  LL2 : Outport
  LL3 : Outport  Port=2
  wires:
  Tank2/1(LL2) -> LL2/1, Tank3/7(LL2)
  Tank3/1(LL3) -> LL3/1, Tank2/7(LL3)
  EB2/1 -> Tank2/6(EB2)
  MR3/1 -> Tank3/4(MR3)
  CT2/1 -> Tank2/1(CT2)
  F2/1 -> Tank2/2(F2)
  E3/1 -> Tank3/3(E3)
  E2/1 -> Tank2/3(E2)
  T2/1 -> Tank2/5(T2)
  CT3/1 -> Tank3/1(CT3)
  F3/1 -> Tank3/2(F3)
  EB3/1 -> Tank3/6(EB3)
  T3/1 -> Tank3/5(T3)
  MR2/1 -> Tank2/4(MR2)

== system c00006M_harness/M093 ==
  note: VALUES
      | ---------------------------------
      | ControlType = 1 | 2 | 3
      | FillTank = 0 | 1
      | EmptyTank = 0 | 1
      | ManualReference between 0 and 1
      | Tempreature between 0 and 100
      | EmergencyButton = 0 | 1
      | LiquidLevel between 0 and 1 (hmax)
  note: Inputs For Tank2
  note: NAMES
      | --------------------------------------------
      | CT1 = ControlType Tank 1
      | F1 = Fill Tank 1
      | E1 = Empty Tank 1
      | MR1 = Manual Reference Tank1
      | T1 = Temperature Tank 1
      | EB1 = Emergency Button Tank 1
      | LL1 = Liquid Level 1
  note: Inputs For Tank3
  note: Inputs For Tank1
  CT2 : Inport
  F2 : Inport  Port=2
  E2 : Inport  Port=3
  MR2 : Inport  Port=4
  T2 : Inport  Port=5
  EB2 : Inport  Port=6
  CT3 : Inport  Port=7
  F3 : Inport  Port=8
  E3 : Inport  Port=9
  MR3 : Inport  Port=10
  T3 : Inport  Port=11
  EB3 : Inport  Port=12
  Tank2 : Subsystem
  Tank3 : Subsystem
  LL2 : Outport
  LL3 : Outport  Port=2
  wires:
  Tank2/1(LL2) -> LL2/1, Tank3/7(LL2)
  Tank3/1(LL3) -> LL3/1, Tank2/7(LL3)
  EB2/1 -> Tank2/6(EB2)
  MR3/1 -> Tank3/4(MR3)
  CT2/1 -> Tank2/1(CT2)
  F2/1 -> Tank2/2(F2)
  E3/1 -> Tank3/3(E3)
  E2/1 -> Tank2/3(E2)
  T2/1 -> Tank2/5(T2)
  CT3/1 -> Tank3/1(CT3)
  F3/1 -> Tank3/2(F3)
  EB3/1 -> Tank3/6(EB3)
  T3/1 -> Tank3/5(T3)
  MR2/1 -> Tank2/4(MR2)

== system c00006M_harness/M094 ==
  note: VALUES
      | ---------------------------------
      | ControlType = 1 | 2 | 3
      | FillTank = 0 | 1
      | EmptyTank = 0 | 1
      | ManualReference between 0 and 1
      | Tempreature between 0 and 100
      | EmergencyButton = 0 | 1
      | LiquidLevel between 0 and 1 (hmax)
  note: Inputs For Tank2
  note: NAMES
      | --------------------------------------------
      | CT1 = ControlType Tank 1
      | F1 = Fill Tank 1
      | E1 = Empty Tank 1
      | MR1 = Manual Reference Tank1
      | T1 = Temperature Tank 1
      | EB1 = Emergency Button Tank 1
      | LL1 = Liquid Level 1
  note: Inputs For Tank3
  note: Inputs For Tank1
  CT2 : Inport
  F2 : Inport  Port=2
  E2 : Inport  Port=3
  MR2 : Inport  Port=4
  T2 : Inport  Port=5
  EB2 : Inport  Port=6
  CT3 : Inport  Port=7
  F3 : Inport  Port=8
  E3 : Inport  Port=9
  MR3 : Inport  Port=10
  T3 : Inport  Port=11
  EB3 : Inport  Port=12
  Tank2 : Subsystem
  Tank3 : Subsystem
  LL2 : Outport
  LL3 : Outport  Port=2
  wires:
  Tank2/1(LL2) -> LL2/1, Tank3/7(LL2)
  Tank3/1(LL3) -> LL3/1, Tank2/7(LL3)
  EB2/1 -> Tank2/6(EB2)
  MR3/1 -> Tank3/4(MR3)
  CT2/1 -> Tank2/1(CT2)
  F2/1 -> Tank2/2(F2)
  E3/1 -> Tank3/3(E3)
  E2/1 -> Tank2/3(E2)
  T2/1 -> Tank2/5(T2)
  CT3/1 -> Tank3/1(CT3)
  F3/1 -> Tank3/2(F3)
  EB3/1 -> Tank3/6(EB3)
  T3/1 -> Tank3/5(T3)
  MR2/1 -> Tank2/4(MR2)

== system c00006M_harness/M095 ==
  note: VALUES
      | ---------------------------------
      | ControlType = 1 | 2 | 3
      | FillTank = 0 | 1
      | EmptyTank = 0 | 1
      | ManualReference between 0 and 1
      | Tempreature between 0 and 100
      | EmergencyButton = 0 | 1
      | LiquidLevel between 0 and 1 (hmax)
  note: Inputs For Tank2
  note: NAMES
      | --------------------------------------------
      | CT1 = ControlType Tank 1
      | F1 = Fill Tank 1
      | E1 = Empty Tank 1
      | MR1 = Manual Reference Tank1
      | T1 = Temperature Tank 1
      | EB1 = Emergency Button Tank 1
      | LL1 = Liquid Level 1
  note: Inputs For Tank3
  note: Inputs For Tank1
  CT2 : Inport
  F2 : Inport  Port=2
  E2 : Inport  Port=3
  MR2 : Inport  Port=4
  T2 : Inport  Port=5
  EB2 : Inport  Port=6
  CT3 : Inport  Port=7
  F3 : Inport  Port=8
  E3 : Inport  Port=9
  MR3 : Inport  Port=10
  T3 : Inport  Port=11
  EB3 : Inport  Port=12
  Tank2 : Subsystem
  Tank3 : Subsystem
  LL2 : Outport
  LL3 : Outport  Port=2
  wires:
  Tank2/1(LL2) -> LL2/1, Tank3/7(LL2)
  Tank3/1(LL3) -> LL3/1, Tank2/7(LL3)
  EB2/1 -> Tank2/6(EB2)
  MR3/1 -> Tank3/4(MR3)
  CT2/1 -> Tank2/1(CT2)
  F2/1 -> Tank2/2(F2)
  E3/1 -> Tank3/3(E3)
  E2/1 -> Tank2/3(E2)
  T2/1 -> Tank2/5(T2)
  CT3/1 -> Tank3/1(CT3)
  F3/1 -> Tank3/2(F3)
  EB3/1 -> Tank3/6(EB3)
  T3/1 -> Tank3/5(T3)
  MR2/1 -> Tank2/4(MR2)

== system c00006M_harness/M096 ==
  note: VALUES
      | ---------------------------------
      | ControlType = 1 | 2 | 3
      | FillTank = 0 | 1
      | EmptyTank = 0 | 1
      | ManualReference between 0 and 1
      | Tempreature between 0 and 100
      | EmergencyButton = 0 | 1
      | LiquidLevel between 0 and 1 (hmax)
  note: Inputs For Tank2
  note: NAMES
      | --------------------------------------------
      | CT1 = ControlType Tank 1
      | F1 = Fill Tank 1
      | E1 = Empty Tank 1
      | MR1 = Manual Reference Tank1
      | T1 = Temperature Tank 1
      | EB1 = Emergency Button Tank 1
      | LL1 = Liquid Level 1
  note: Inputs For Tank3
  note: Inputs For Tank1
  CT2 : Inport
  F2 : Inport  Port=2
  E2 : Inport  Port=3
  MR2 : Inport  Port=4
  T2 : Inport  Port=5
  EB2 : Inport  Port=6
  CT3 : Inport  Port=7
  F3 : Inport  Port=8
  E3 : Inport  Port=9
  MR3 : Inport  Port=10
  T3 : Inport  Port=11
  EB3 : Inport  Port=12
  Tank2 : Subsystem
  Tank3 : Subsystem
  LL2 : Outport
  LL3 : Outport  Port=2
  wires:
  Tank2/1(LL2) -> LL2/1, Tank3/7(LL2)
  Tank3/1(LL3) -> LL3/1, Tank2/7(LL3)
  EB2/1 -> Tank2/6(EB2)
  MR3/1 -> Tank3/4(MR3)
  CT2/1 -> Tank2/1(CT2)
  F2/1 -> Tank2/2(F2)
  E3/1 -> Tank3/3(E3)
  E2/1 -> Tank2/3(E2)
  T2/1 -> Tank2/5(T2)
  CT3/1 -> Tank3/1(CT3)
  F3/1 -> Tank3/2(F3)
  EB3/1 -> Tank3/6(EB3)
  T3/1 -> Tank3/5(T3)
  MR2/1 -> Tank2/4(MR2)

== system c00006M_harness/M097 ==
  note: VALUES
      | ---------------------------------
      | ControlType = 1 | 2 | 3
      | FillTank = 0 | 1
      | EmptyTank = 0 | 1
      | ManualReference between 0 and 1
      | Tempreature between 0 and 100
      | EmergencyButton = 0 | 1
      | LiquidLevel between 0 and 1 (hmax)
  note: Inputs For Tank2
  note: NAMES
      | --------------------------------------------
      | CT1 = ControlType Tank 1
      | F1 = Fill Tank 1
      | E1 = Empty Tank 1
      | MR1 = Manual Reference Tank1
      | T1 = Temperature Tank 1
      | EB1 = Emergency Button Tank 1
      | LL1 = Liquid Level 1
  note: Inputs For Tank3
  note: Inputs For Tank1
  CT2 : Inport
  F2 : Inport  Port=2
  E2 : Inport  Port=3
  MR2 : Inport  Port=4
  T2 : Inport  Port=5
  EB2 : Inport  Port=6
  CT3 : Inport  Port=7
  F3 : Inport  Port=8
  E3 : Inport  Port=9
  MR3 : Inport  Port=10
  T3 : Inport  Port=11
  EB3 : Inport  Port=12
  Tank2 : Subsystem
  Tank3 : Subsystem
  LL2 : Outport
  LL3 : Outport  Port=2
  wires:
  Tank2/1(LL2) -> LL2/1, Tank3/7(LL2)
  Tank3/1(LL3) -> LL3/1, Tank2/7(LL3)
  EB2/1 -> Tank2/6(EB2)
  MR3/1 -> Tank3/4(MR3)
  CT2/1 -> Tank2/1(CT2)
  F2/1 -> Tank2/2(F2)
  E3/1 -> Tank3/3(E3)
  E2/1 -> Tank2/3(E2)
  T2/1 -> Tank2/5(T2)
  CT3/1 -> Tank3/1(CT3)
  F3/1 -> Tank3/2(F3)
  EB3/1 -> Tank3/6(EB3)
  T3/1 -> Tank3/5(T3)
  MR2/1 -> Tank2/4(MR2)

== system c00006M_harness/M098 ==
  note: VALUES
      | ---------------------------------
      | ControlType = 1 | 2 | 3
      | FillTank = 0 | 1
      | EmptyTank = 0 | 1
      | ManualReference between 0 and 1
      | Tempreature between 0 and 100
      | EmergencyButton = 0 | 1
      | LiquidLevel between 0 and 1 (hmax)
  note: Inputs For Tank2
  note: NAMES
      | --------------------------------------------
      | CT1 = ControlType Tank 1
      | F1 = Fill Tank 1
      | E1 = Empty Tank 1
      | MR1 = Manual Reference Tank1
      | T1 = Temperature Tank 1
      | EB1 = Emergency Button Tank 1
      | LL1 = Liquid Level 1
  note: Inputs For Tank3
  note: Inputs For Tank1
  CT2 : Inport
  F2 : Inport  Port=2
  E2 : Inport  Port=3
  MR2 : Inport  Port=4
  T2 : Inport  Port=5
  EB2 : Inport  Port=6
  CT3 : Inport  Port=7
  F3 : Inport  Port=8
  E3 : Inport  Port=9
  MR3 : Inport  Port=10
  T3 : Inport  Port=11
  EB3 : Inport  Port=12
  Tank2 : Subsystem
  Tank3 : Subsystem
  LL2 : Outport
  LL3 : Outport  Port=2
  wires:
  Tank2/1(LL2) -> LL2/1, Tank3/7(LL2)
  Tank3/1(LL3) -> LL3/1, Tank2/7(LL3)
  EB2/1 -> Tank2/6(EB2)
  MR3/1 -> Tank3/4(MR3)
  CT2/1 -> Tank2/1(CT2)
  F2/1 -> Tank2/2(F2)
  E3/1 -> Tank3/3(E3)
  E2/1 -> Tank2/3(E2)
  T2/1 -> Tank2/5(T2)
  CT3/1 -> Tank3/1(CT3)
  F3/1 -> Tank3/2(F3)
  EB3/1 -> Tank3/6(EB3)
  T3/1 -> Tank3/5(T3)
  MR2/1 -> Tank2/4(MR2)

== system c00006M_harness/M099 ==
  note: VALUES
      | ---------------------------------
      | ControlType = 1 | 2 | 3
      | FillTank = 0 | 1
      | EmptyTank = 0 | 1
      | ManualReference between 0 and 1
      | Tempreature between 0 and 100
      | EmergencyButton = 0 | 1
      | LiquidLevel between 0 and 1 (hmax)
  note: Inputs For Tank2
  note: NAMES
      | --------------------------------------------
      | CT1 = ControlType Tank 1
      | F1 = Fill Tank 1
      | E1 = Empty Tank 1
      | MR1 = Manual Reference Tank1
      | T1 = Temperature Tank 1
      | EB1 = Emergency Button Tank 1
      | LL1 = Liquid Level 1
  note: Inputs For Tank3
  note: Inputs For Tank1
  CT2 : Inport
  F2 : Inport  Port=2
  E2 : Inport  Port=3
  MR2 : Inport  Port=4
  T2 : Inport  Port=5
  EB2 : Inport  Port=6
  CT3 : Inport  Port=7
  F3 : Inport  Port=8
  E3 : Inport  Port=9
  MR3 : Inport  Port=10
  T3 : Inport  Port=11
  EB3 : Inport  Port=12
  Tank2 : Subsystem
  Tank3 : Subsystem
  LL2 : Outport
  LL3 : Outport  Port=2
  wires:
  Tank2/1(LL2) -> LL2/1, Tank3/7(LL2)
  Tank3/1(LL3) -> LL3/1, Tank2/7(LL3)
  EB2/1 -> Tank2/6(EB2)
  MR3/1 -> Tank3/4(MR3)
  CT2/1 -> Tank2/1(CT2)
  F2/1 -> Tank2/2(F2)
  E3/1 -> Tank3/3(E3)
  E2/1 -> Tank2/3(E2)
  T2/1 -> Tank2/5(T2)
  CT3/1 -> Tank3/1(CT3)
  F3/1 -> Tank3/2(F3)
  EB3/1 -> Tank3/6(EB3)
  T3/1 -> Tank3/5(T3)
  MR2/1 -> Tank2/4(MR2)

== system c00006M_harness/M100 ==
  note: VALUES
      | ---------------------------------
      | ControlType = 1 | 2 | 3
      | FillTank = 0 | 1
      | EmptyTank = 0 | 1
      | ManualReference between 0 and 1
      | Tempreature between 0 and 100
      | EmergencyButton = 0 | 1
      | LiquidLevel between 0 and 1 (hmax)
  note: Inputs For Tank2
  note: NAMES
      | --------------------------------------------
      | CT1 = ControlType Tank 1
      | F1 = Fill Tank 1
      | E1 = Empty Tank 1
      | MR1 = Manual Reference Tank1
      | T1 = Temperature Tank 1
      | EB1 = Emergency Button Tank 1
      | LL1 = Liquid Level 1
  note: Inputs For Tank3
  note: Inputs For Tank1
  CT2 : Inport
  F2 : Inport  Port=2
  E2 : Inport  Port=3
  MR2 : Inport  Port=4
  T2 : Inport  Port=5
  EB2 : Inport  Port=6
  CT3 : Inport  Port=7
  F3 : Inport  Port=8
  E3 : Inport  Port=9
  MR3 : Inport  Port=10
  T3 : Inport  Port=11
  EB3 : Inport  Port=12
  Tank2 : Subsystem
  Tank3 : Subsystem
  LL2 : Outport
  LL3 : Outport  Port=2
  wires:
  Tank2/1(LL2) -> LL2/1, Tank3/7(LL2)
  Tank3/1(LL3) -> LL3/1, Tank2/7(LL3)
  EB2/1 -> Tank2/6(EB2)
  MR3/1 -> Tank3/4(MR3)
  CT2/1 -> Tank2/1(CT2)
  F2/1 -> Tank2/2(F2)
  E3/1 -> Tank3/3(E3)
  E2/1 -> Tank2/3(E2)
  T2/1 -> Tank2/5(T2)
  CT3/1 -> Tank3/1(CT3)
  F3/1 -> Tank3/2(F3)
  EB3/1 -> Tank3/6(EB3)
  T3/1 -> Tank3/5(T3)
  MR2/1 -> Tank2/4(MR2)

== system c00006M_harness/M101 ==
  note: VALUES
      | ---------------------------------
      | ControlType = 1 | 2 | 3
      | FillTank = 0 | 1
      | EmptyTank = 0 | 1
      | ManualReference between 0 and 1
      | Tempreature between 0 and 100
      | EmergencyButton = 0 | 1
      | LiquidLevel between 0 and 1 (hmax)
  note: Inputs For Tank2
  note: NAMES
      | --------------------------------------------
      | CT1 = ControlType Tank 1
      | F1 = Fill Tank 1
      | E1 = Empty Tank 1
      | MR1 = Manual Reference Tank1
      | T1 = Temperature Tank 1
      | EB1 = Emergency Button Tank 1
      | LL1 = Liquid Level 1
  note: Inputs For Tank3
  note: Inputs For Tank1
  CT2 : Inport
  F2 : Inport  Port=2
  E2 : Inport  Port=3
  MR2 : Inport  Port=4
  T2 : Inport  Port=5
  EB2 : Inport  Port=6
  CT3 : Inport  Port=7
  F3 : Inport  Port=8
  E3 : Inport  Port=9
  MR3 : Inport  Port=10
  T3 : Inport  Port=11
  EB3 : Inport  Port=12
  Tank2 : Subsystem
  Tank3 : Subsystem
  LL2 : Outport
  LL3 : Outport  Port=2
  wires:
  Tank2/1(LL2) -> LL2/1, Tank3/7(LL2)
  Tank3/1(LL3) -> LL3/1, Tank2/7(LL3)
  EB2/1 -> Tank2/6(EB2)
  MR3/1 -> Tank3/4(MR3)
  CT2/1 -> Tank2/1(CT2)
  F2/1 -> Tank2/2(F2)
  E3/1 -> Tank3/3(E3)
  E2/1 -> Tank2/3(E2)
  T2/1 -> Tank2/5(T2)
  CT3/1 -> Tank3/1(CT3)
  F3/1 -> Tank3/2(F3)
  EB3/1 -> Tank3/6(EB3)
  T3/1 -> Tank3/5(T3)
  MR2/1 -> Tank2/4(MR2)

== system c00006M_harness/M102 ==
  note: VALUES
      | ---------------------------------
      | ControlType = 1 | 2 | 3
      | FillTank = 0 | 1
      | EmptyTank = 0 | 1
      | ManualReference between 0 and 1
      | Tempreature between 0 and 100
      | EmergencyButton = 0 | 1
      | LiquidLevel between 0 and 1 (hmax)
  note: Inputs For Tank2
  note: NAMES
      | --------------------------------------------
      | CT1 = ControlType Tank 1
      | F1 = Fill Tank 1
      | E1 = Empty Tank 1
      | MR1 = Manual Reference Tank1
      | T1 = Temperature Tank 1
      | EB1 = Emergency Button Tank 1
      | LL1 = Liquid Level 1
  note: Inputs For Tank3
  note: Inputs For Tank1
  CT2 : Inport
  F2 : Inport  Port=2
  E2 : Inport  Port=3
  MR2 : Inport  Port=4
  T2 : Inport  Port=5
  EB2 : Inport  Port=6
  CT3 : Inport  Port=7
  F3 : Inport  Port=8
  E3 : Inport  Port=9
  MR3 : Inport  Port=10
  T3 : Inport  Port=11
  EB3 : Inport  Port=12
  Tank2 : Subsystem
  Tank3 : Subsystem
  LL2 : Outport
  LL3 : Outport  Port=2
  wires:
  Tank2/1(LL2) -> LL2/1, Tank3/7(LL2)
  Tank3/1(LL3) -> LL3/1, Tank2/7(LL3)
  EB2/1 -> Tank2/6(EB2)
  MR3/1 -> Tank3/4(MR3)
  CT2/1 -> Tank2/1(CT2)
  F2/1 -> Tank2/2(F2)
  E3/1 -> Tank3/3(E3)
  E2/1 -> Tank2/3(E2)
  T2/1 -> Tank2/5(T2)
  CT3/1 -> Tank3/1(CT3)
  F3/1 -> Tank3/2(F3)
  EB3/1 -> Tank3/6(EB3)
  T3/1 -> Tank3/5(T3)
  MR2/1 -> Tank2/4(MR2)

== system c00006M_harness/M103 ==
  note: VALUES
      | ---------------------------------
      | ControlType = 1 | 2 | 3
      | FillTank = 0 | 1
      | EmptyTank = 0 | 1
      | ManualReference between 0 and 1
      | Tempreature between 0 and 100
      | EmergencyButton = 0 | 1
      | LiquidLevel between 0 and 1 (hmax)
  note: Inputs For Tank2
  note: NAMES
      | --------------------------------------------
      | CT1 = ControlType Tank 1
      | F1 = Fill Tank 1
      | E1 = Empty Tank 1
      | MR1 = Manual Reference Tank1
      | T1 = Temperature Tank 1
      | EB1 = Emergency Button Tank 1
      | LL1 = Liquid Level 1
  note: Inputs For Tank3
  note: Inputs For Tank1
  CT2 : Inport
  F2 : Inport  Port=2
  E2 : Inport  Port=3
  MR2 : Inport  Port=4
  T2 : Inport  Port=5
  EB2 : Inport  Port=6
  CT3 : Inport  Port=7
  F3 : Inport  Port=8
  E3 : Inport  Port=9
  MR3 : Inport  Port=10
  T3 : Inport  Port=11
  EB3 : Inport  Port=12
  Tank2 : Subsystem
  Tank3 : Subsystem
  LL2 : Outport
  LL3 : Outport  Port=2
  wires:
  Tank2/1(LL2) -> LL2/1, Tank3/7(LL2)
  Tank3/1(LL3) -> LL3/1, Tank2/7(LL3)
  EB2/1 -> Tank2/6(EB2)
  MR3/1 -> Tank3/4(MR3)
  CT2/1 -> Tank2/1(CT2)
  F2/1 -> Tank2/2(F2)
  E3/1 -> Tank3/3(E3)
  E2/1 -> Tank2/3(E2)
  T2/1 -> Tank2/5(T2)
  CT3/1 -> Tank3/1(CT3)
  F3/1 -> Tank3/2(F3)
  EB3/1 -> Tank3/6(EB3)
  T3/1 -> Tank3/5(T3)
  MR2/1 -> Tank2/4(MR2)

== system c00006M_harness/M104 ==
  note: VALUES
      | ---------------------------------
      | ControlType = 1 | 2 | 3
      | FillTank = 0 | 1
      | EmptyTank = 0 | 1
      | ManualReference between 0 and 1
      | Tempreature between 0 and 100
      | EmergencyButton = 0 | 1
      | LiquidLevel between 0 and 1 (hmax)
  note: Inputs For Tank2
  note: NAMES
      | --------------------------------------------
      | CT1 = ControlType Tank 1
      | F1 = Fill Tank 1
      | E1 = Empty Tank 1
      | MR1 = Manual Reference Tank1
      | T1 = Temperature Tank 1
      | EB1 = Emergency Button Tank 1
      | LL1 = Liquid Level 1
  note: Inputs For Tank3
  note: Inputs For Tank1
  CT2 : Inport
  F2 : Inport  Port=2
  E2 : Inport  Port=3
  MR2 : Inport  Port=4
  T2 : Inport  Port=5
  EB2 : Inport  Port=6
  CT3 : Inport  Port=7
  F3 : Inport  Port=8
  E3 : Inport  Port=9
  MR3 : Inport  Port=10
  T3 : Inport  Port=11
  EB3 : Inport  Port=12
  Tank2 : Subsystem
  Tank3 : Subsystem
  LL2 : Outport
  LL3 : Outport  Port=2
  wires:
  Tank2/1(LL2) -> LL2/1, Tank3/7(LL2)
  Tank3/1(LL3) -> LL3/1, Tank2/7(LL3)
  EB2/1 -> Tank2/6(EB2)
  MR3/1 -> Tank3/4(MR3)
  CT2/1 -> Tank2/1(CT2)
  F2/1 -> Tank2/2(F2)
  E3/1 -> Tank3/3(E3)
  E2/1 -> Tank2/3(E2)
  T2/1 -> Tank2/5(T2)
  CT3/1 -> Tank3/1(CT3)
  F3/1 -> Tank3/2(F3)
  EB3/1 -> Tank3/6(EB3)
  T3/1 -> Tank3/5(T3)
  MR2/1 -> Tank2/4(MR2)
